simulink model "lin_hover_sim"  (R2025b)
settings: Solver=VariableStepAuto  StartTime=0.0  StopTime=t_sim  RelTol=1e-6  AbsTol=1e-6
values from neighbouring files (symbols this model uses):
  A = zeros(12,12)    [lin_hover.m]
  A_kfd = sys_kf_d.A    [lin_hover.m]
  Aomega = 1.00*Aref    (= 0.486439179934)    [lin_hover.m]    (also in non_lin_sim.m)
  Ax = 0.50*Aref    (= 0.243219589967)    [lin_hover.m]    (also in non_lin_sim.m)
  Ay = 0.50*Aref    (= 0.243219589967)    [lin_hover.m]    (also in non_lin_sim.m)
  Az = 0.35*Aref    (= 0.170253712977)    [lin_hover.m]    (also in non_lin_sim.m)
  B = zeros(12,4)    [lin_hover.m]
  B_kfd = sys_kf_d.B    [lin_hover.m]
  C11 = 4.58e-4    (= 0.000458)    [lin_hover.m]    (also in non_lin_sim.m)
  C21 = -.562    (= -0.562)    [lin_hover.m]    (also in non_lin_sim.m)
  CDw = 1.0    (= 1)    [lin_hover.m]    (also in non_lin_sim.m)
  CDx = 1.0    (= 1)    [lin_hover.m]    (also in non_lin_sim.m)
  CDy = 1.0    (= 1)    [lin_hover.m]    (also in non_lin_sim.m)
  CDz = 1.0    (= 1)    [lin_hover.m]    (also in non_lin_sim.m)
  g = 9.81    [lin_hover.m]    (also in non_lin_sim.m)
  Ix = I(1,1)    [lin_hover.m]    (also in non_lin_sim.m)
  Iy = I(2,2)    [lin_hover.m]    (also in non_lin_sim.m)
  Iz = I(3,3)    [lin_hover.m]    (also in non_lin_sim.m)
  k_tau = 0.00    (= 0)    [lin_hover.m]    (also in non_lin_sim.m)
  m = 0.110    (= 0.11)    [lin_hover.m]    (also in non_lin_sim.m)
  max_pot = 1950    [lin_hover.m]
  noise_true = 1    [lin_hover.m]
  pitch_D = 0    [lin_hover.m]
  pitch_I = 0.005*Iy/Ix    [lin_hover.m]
  pitch_P = 0.022*Iy/Ix    [lin_hover.m]
  rho = 1.225    [lin_hover.m]    (also in non_lin_sim.m)
  roll_D = 0    [lin_hover.m]
  roll_I = 0.005    [lin_hover.m]
  roll_P = 0.022    [lin_hover.m]
  S = 0.11    [lin_hover.m]    (also in non_lin_sim.m)
  seed = 23341    [lin_hover.m]
  sim_fidelity = 'high'    [lin_hover.m]
  strength = 50    [lin_hover.m]
  tau_wing = 0.1/2.2    (= 0.0454545454545)    [lin_hover.m]
  Ts = 1/fs    (= 0.00025)    [lin_hover.m]
  u0 = (m*g/4 - C21)/C11    (= 1816.10262009)    [lin_hover.m]
  X0 = zeros([12,1])    [lin_hover.m]
  Xref = zeros([12,1])    [lin_hover.m]
  Xu = rho*CDx*Ax*v_ref    (= 0.148971998855)    [lin_hover.m]    (also in non_lin_sim.m)
  yaw_D = 0    [lin_hover.m]
  yaw_I = 0.001    [lin_hover.m]
  yaw_P = 0.001    [lin_hover.m]
  Yv = rho*CDy*Ay*v_ref    (= 0.148971998855)    [lin_hover.m]    (also in non_lin_sim.m)
  Zw = rho*CDz*Az*w_ref    (= 0.104280399198)    [lin_hover.m]    (also in non_lin_sim.m)
undefined symbols (not defined in the file or in its folder): accel, C_kf, D_kf, DiscIntNeverNeededParam, Discrete, dspblkCoreblockFVToolHelper, gcbh, gyro, mahoney, R_kf, Time, x_kf0
libraries: slpidlib x5, simulink_extras x5, simulink x3, ctrlSharedLib x1
settings Model: Creator=bmatt  LastModifiedBy=bmatt
settings DebuggingCC: SignalInfNanChecking=error  SignalRangeChecking=error

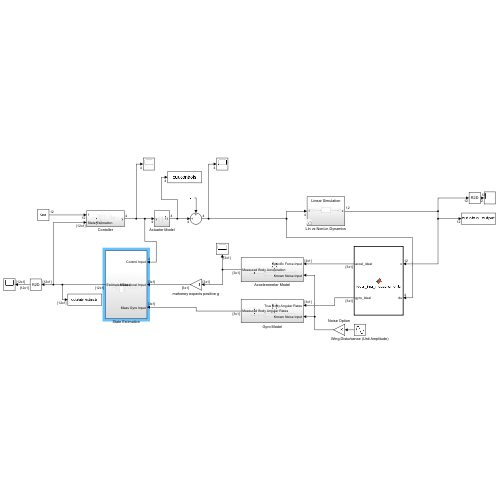
[thumbnail: Simulink's stored preview of the top-level diagram]
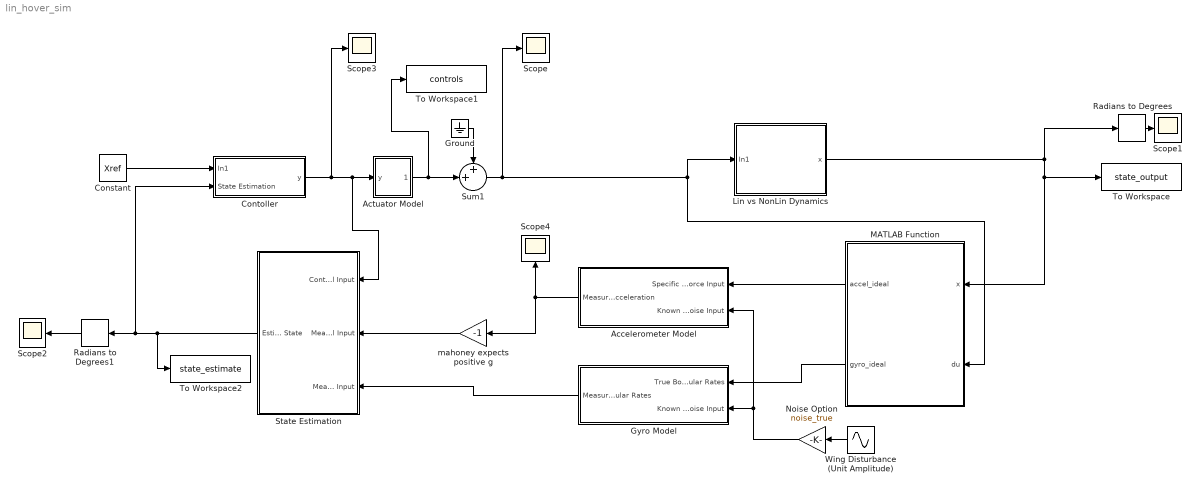
== system lin_hover_sim ==
  Accelerometer Model : Subsystem
  Actuator Model : Subsystem
  Constant : Constant  Value=Xref  SampleTime=-1
  Contoller : Subsystem
  Ground : Ground
  Gyro Model : Subsystem
  Lin vs NonLin Dynamics : Subsystem  Variant=on
  MATLAB Function : MATLAB Function  TreatAsAtomicUnit=on
  Noise Option : Gain  Gain=noise_true
  Radians to Degrees : simulink_extras/Transformations/Radians to Degrees
  Radians to Degrees1 : simulink_extras/Transformations/Radians to Degrees
  Scope{,1..4} (5 alike) : Scope
      Scope settings: ActiveDisplayYMinimum=-18.295353079019556  ActiveDisplayYMaximum=14.608808990960183
      Scope1 settings: ActiveDisplayYMinimum=-57.493316939596269  ActiveDisplayYMaximum=14.428367766901045
      Scope2 settings: ActiveDisplayYMinimum=-37.103950229220729  ActiveDisplayYMaximum=16.0841911942195  DataLoggingVariableName=ScopeData2
      Scope3 settings: ActiveDisplayYMinimum=-1  ActiveDisplayYMaximum=1  DataLoggingVariableName=ScopeData9
      Scope4 settings: ActiveDisplayYMinimum=-26.796825567144111  ActiveDisplayYMaximum=14.82950437821362  DataLoggingVariableName=ScopeData10
  State Estimation : Subsystem
  Sum1 : Sum  Inputs=++|
  To Workspace : ToWorkspace  VariableName=state_output  SaveFormat=Structure With Time  SampleTime=-1
  To Workspace1 : ToWorkspace  VariableName=controls  SaveFormat=Structure With Time  SampleTime=-1
  To Workspace2 : ToWorkspace  VariableName=state_estimate  SaveFormat=Structure With Time  SampleTime=-1
  Wing Disturbance (Unit Amplitude) : Sin  Frequency=2*pi*24  SampleTime=0
  mahoney expects positive g : Gain  Gain=-1
  wires:
  Sum1/1 -> Scope/1, Lin vs NonLin Dynamics/1(In1), MATLAB Function/2(du)
  Constant/1 -> Contoller/1(In1)
  Contoller/1(y) -> Actuator Model/1(y), State Estimation/1(Control Input), Scope3/1
  Actuator Model/1(Out1) -> Sum1/2, To Workspace1/1
  State Estimation/1(Estimated State) -> To Workspace2/1, Contoller/2(State Estimation), Radians to Degrees1/1
  Ground/1 -> Sum1/1
  Radians to Degrees/1 -> Scope1/1
  Radians to Degrees1/1 -> Scope2/1
  Accelerometer Model/1(Measured Body Acceleration) -> mahoney expects positive g/1, Scope4/1
  Gyro Model/1(Measured Body Angular Rates) -> State Estimation/3(Meas Gyro Input)
  MATLAB Function/1(accel_ideal) -> Accelerometer Model/1(Specific Force Input)
  MATLAB Function/2(gyro_ideal) -> Gyro Model/1(True Body Angular Rates)
  mahoney expects positive g/1 -> State Estimation/2(Meas Accel Input)
  Wing Disturbance (Unit Amplitude)/1 -> Noise Option/1
  Noise Option/1 -> Accelerometer Model/2(Known Noise Input), Gyro Model/2(Known Noise Input)
  Lin vs NonLin Dynamics/1(x) -> To Workspace/1, MATLAB Function/1(x), Radians to Degrees/1

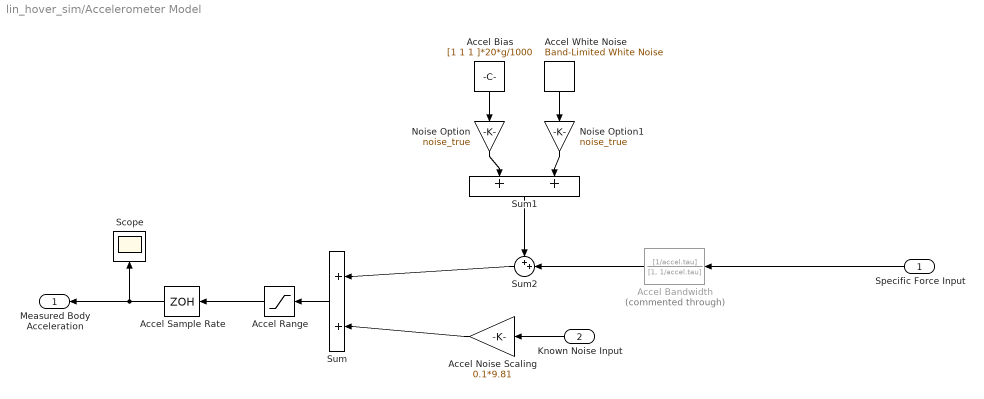
== system lin_hover_sim/Accelerometer Model ==
  Specific Force Input : Inport
  Known Noise Input : Inport  Port=2
  Accel White Noise : simulink/Sources/Band-Limited White Noise  Cov=[1 1 1]*((0.16*9.81/1000)*sqrt(740))^2  Ts=1/1600  seed=[seed]
  Accel Bandwidth : DiscreteTransferFcn  Commented=through  LoadFcn=dspblkCoreblockFVToolHelper(gcbh,'load');  Numerator=[1/accel.tau]  Denominator=[1, 1/accel.tau]
      settings: CopyFcn=dspblkCoreblockFVToolHelper(gcbh,'copy');  DeleteFcn=dspblkCoreblockFVToolHelper(gcbh,'close');  ModelCloseFcn=dspblkCoreblockFVToolHelper(gcbh,'close');  PreSaveFcn=dspblkCoreblockFVToolHelper(gcbh,'presave');  PostSaveFcn=dspblkCoreblockFVToolHelper(gcbh,'postsave');  CloseFcn=dspblkCoreblockFVToolHelper(gcbh,'close');
  Accel Bias : Constant  Value=[1 1 1 ]*20*g/1000  SampleTime=1/1600
  Accel Noise Scaling : Gain  Gain=0.1*9.81
  Accel Range : Saturate  UpperLimit=4*9.81  LowerLimit=-4*9.81
  Accel Sample Rate : ZeroOrderHold  SampleTime=1/1600
  Noise Option : Gain  Gain=noise_true
  Noise Option1 : Gain  Gain=noise_true
  Scope : Scope
      settings: ActiveDisplayYMinimum=-33.285329290238963  ActiveDisplayYMaximum=9.7506326968606309  DataLoggingVariableName=ScopeData13
  Sum : Sum  Inputs=+|+
  Sum1 : Sum  Inputs=+|+
  Sum2 : Sum  Inputs=++|
  Measured Body Acceleration : Outport
  wires:
  Sum/1 -> Accel Range/1
  Sum2/1 -> Sum/1
  Accel Sample Rate/1 -> Scope/1, Measured Body Acceleration/1
  Known Noise Input/1 -> Accel Noise Scaling/1
  Accel Bandwidth/1 -> Sum2/2
  Specific Force Input/1 -> Accel Bandwidth/1
  Sum1/1 -> Sum2/1
  Accel Noise Scaling/1 -> Sum/2
  Accel Range/1 -> Accel Sample Rate/1
  Noise Option/1 -> Sum1/1
  Accel Bias/1 -> Noise Option/1
  Noise Option1/1 -> Sum1/2
  Accel White Noise/1 -> Noise Option1/1

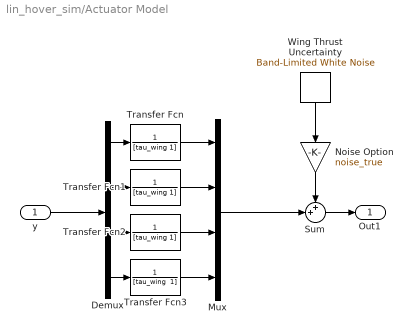
== system lin_hover_sim/Actuator Model ==
  y : Inport
  Demux : Demux
  Mux : Mux
  Noise Option : Gain  Gain=noise_true
  Sum : Sum  Inputs=++|
  Transfer Fcn : TransferFcn  Denominator=[tau_wing 1]
  Transfer Fcn1 : TransferFcn  Denominator=[tau_wing 1]
  Transfer Fcn2 : TransferFcn  Denominator=[tau_wing 1]
  Transfer Fcn3 : TransferFcn  Denominator="[tau_wing  1]"
  Wing Thrust Uncertainty : simulink/Sources/Band-Limited White Noise  Cov=1*[0.000001566122567;0.000001566122567;0.000001566122567;0.000001566122567]  Ts=Ts  seed=[seed]
  Out1 : Outport
  wires:
  Demux/4 -> Transfer Fcn3/1
  Demux/1 -> Transfer Fcn/1
  Demux/2 -> Transfer Fcn1/1
  Demux/3 -> Transfer Fcn2/1
  Transfer Fcn/1 -> Mux/1
  Transfer Fcn1/1 -> Mux/2
  Transfer Fcn2/1 -> Mux/3
  Transfer Fcn3/1 -> Mux/4
  y/1 -> Demux/1
  Sum/1 -> Out1/1
  Mux/1 -> Sum/2
  Wing Thrust Uncertainty/1 -> Noise Option/1
  Noise Option/1 -> Sum/1

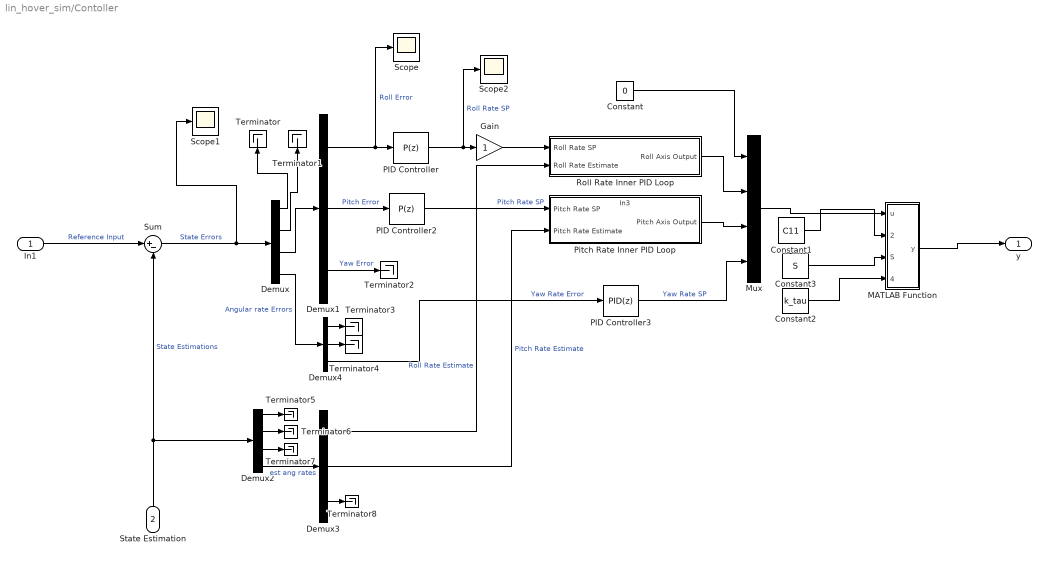
== system lin_hover_sim/Contoller ==
  In1 : Inport
  State Estimation : Inport  Port=2
  Constant : Constant  Value=0
  Constant1 : Constant  Value=C11
  Constant2 : Constant  Value=k_tau
  Constant3 : Constant  Value=S
  Demux : Demux  Outputs=[3 3 3 3]
  Demux1 : Demux  Outputs=[1 1 1]
  Demux2 : Demux  Outputs=[3 3 3 3]
  Demux3 : Demux  Outputs=[1 1 1]
  Demux4 : Demux  Outputs=[1 1 1]
  Gain : Gain
  MATLAB Function : MATLAB Function  TreatAsAtomicUnit=on
  Mux : Mux
  PID Controller : slpidlib/PID Controller  Controller=P  Form=Parallel  TimeDomain=Discrete-time  UseExternalTs=off  SampleTime=Ts  IntegratorMethod=Forward Euler  FilterMethod=Forward Euler  ControllerParametersSource=internal  P=strength/10  I=194.232873086371  UseKiTs=off  D=-0.0894221705749344  UseExternalDerivativeSource=off  N=55.5911819026225  UseFilter=on  TunerSelectOption=Frequency Response Based  InitialConditionSource=internal  InitialConditionForIntegrator=Xref(7) - X0(7)  InitialConditionForFilter=0  DifferentiatorICPrevScaledInput=0  ExternalReset=none  TrackingMode=off  Kt=1  LimitOutput=on  SatLimitsSource=internal  UpperSaturationLimit=3.5  LowerSaturationLimit=-3.5  LinearizeAsGain=on  AntiWindupMode=external  Kb=1  LimitIntegrator=off  UpperIntegratorSaturationLimit=inf  LowerIntegratorSaturationLimit=-inf  POutMin=[]  POutMax=[]  IOutMin=[]  IOutMax=[]  DOutMin=[]  DOutMax=[]  NOutMin=[]  NOutMax=[]  SumOutMin=[]  SumOutMax=[]  SaturationOutMin=[]  SaturationOutMax=[]  PParamMin=[]  PParamMax=[]  IParamMin=[]  IParamMax=[]  DParamMin=[]  DParamMax=[]  NParamMin=[]  NParamMax=[]  KbParamMin=[]  KbParamMax=[]  KtParamMin=[]  KtParamMax=[]  KbOutMin=[]  KbOutMax=[]  KtOutMin=[]  KtOutMax=[]  IntegratorOutMin=[]  IntegratorOutMax=[]  FilterOutMin=[]  FilterOutMax=[]  SumI1OutMin=[]  SumI1OutMax=[]  SumI2OutMin=[]  SumI2OutMax=[]  SumI3OutMin=[]  SumI3OutMax=[]  SumI4OutMin=[]  SumI4OutMax=[]  SumDOutMin=[]  SumDOutMax=[]  DifferentiatorOutMin=[]  DifferentiatorOutMax=[]  FilterDiffOutCoefMin=[]  FilterDiffOutCoefMax=[]  ReciprocalOutMin=[]  ReciprocalOutMax=[]  SumDenOutMin=[]  SumDenOutMax=[]  SumNumOutMin=[]  SumNumOutMax=[]  DivideOutMin=[]  DivideOutMax=[]  UdiffTsProdOutMin=[]  UdiffTsProdOutMax=[]  NTsProdOutMin=[]  NTsProdOutMax=[]  UintegralTsProdOutMin=[]  UintegralTsProdOutMax=[]  UngainTsProdOutMin=[]  UngainTsProdOutMax=[]  ClampingZeroOutDataTypeStr=Inherit: Inherit via back propagation  ClampingZeroOutMin=[]  ClampingZeroOutMax=[]  FilterDenConstantOutDataTypeStr=Inherit: Inherit via back propagation  FilterDenConstantOutMin=[]  FilterDenConstantOutMax=[]  PCopyOutDataTypeStr=Inherit: Inherit via back propagation  PCopyOutMin=[]  PCopyOutMax=[]  NCopyOutDataTypeStr=Inherit: Inherit via back propagation  NCopyOutMin=[]  NCopyOutMax=[]  IntegratorContinuousStateAttributes=''  IntegratorStateMustResolveToSignalObject=off  IntegratorRTWStateStorageClass=Auto  FilterContinuousStateAttributes=''  FilterStateMustResolveToSignalObject=off  FilterRTWStateStorageClass=Auto  ParallelPVariant=InternalParameters  IdealPVariant=Disabled  IVariant=Disabled  DVariant=Disabled  IntegratorVariant=Disabled  SatVariant=Enabled  AWVariant=Disabled  PCopyVariant=Disabled  TRVariant=Disabled  FdbkBlocksVariant=Forward  IdealPFdbkVariant=Disabled  SatFdbkVariant=Disabled  DerivativeFilterVariant=Disabled  NVariant=Disabled  NCopyVariant=Disabled_SignalSpec  FilterICVariant=Disabled  IntegratorICVariant=Disabled  ExternalResetVariant=Disabled  TRSumVariant=Passthrough  SumFdbkVariant=Disabled  SumVariant=Passthrough_P  TsampFilterVariant=InternalTs  TsampNgainVariant=Passthrough  TsampIntegralVariant=Disabled_SignalSpec  ExternalSaturationOutDataTypeStr=Inherit: Same as second input  DerivativeSourceVariant=Disabled  PreIntVariant=InternalPreInt
  PID Controller2 : slpidlib/PID Controller  Controller=P  Form=Parallel  TimeDomain=Discrete-time  UseExternalTs=off  SampleTime=Ts  IntegratorMethod=Forward Euler  FilterMethod=Forward Euler  ControllerParametersSource=internal  P=strength/10  I=0.287608182877056  UseKiTs=off  D=0  UseExternalDerivativeSource=off  N=100  UseFilter=on  TunerSelectOption=Transfer Function Based (PID Tuner App)  InitialConditionSource=internal  InitialConditionForIntegrator=Xref(8) - X0(8)  InitialConditionForFilter=0  DifferentiatorICPrevScaledInput=0  ExternalReset=none  TrackingMode=off  Kt=1  LimitOutput=on  SatLimitsSource=internal  UpperSaturationLimit=3.5  LowerSaturationLimit=-3.5  LinearizeAsGain=off  AntiWindupMode=none  Kb=1  LimitIntegrator=off  UpperIntegratorSaturationLimit=inf  LowerIntegratorSaturationLimit=-inf  POutMin=[]  POutMax=[]  IOutMin=[]  IOutMax=[]  DOutMin=[]  DOutMax=[]  NOutMin=[]  NOutMax=[]  SumOutMin=[]  SumOutMax=[]  SaturationOutMin=[]  SaturationOutMax=[]  PParamMin=[]  PParamMax=[]  IParamMin=[]  IParamMax=[]  DParamMin=[]  DParamMax=[]  NParamMin=[]  NParamMax=[]  KbParamMin=[]  KbParamMax=[]  KtParamMin=[]  KtParamMax=[]  KbOutMin=[]  KbOutMax=[]  KtOutMin=[]  KtOutMax=[]  IntegratorOutMin=[]  IntegratorOutMax=[]  FilterOutMin=[]  FilterOutMax=[]  SumI1OutMin=[]  SumI1OutMax=[]  SumI2OutMin=[]  SumI2OutMax=[]  SumI3OutMin=[]  SumI3OutMax=[]  SumI4OutMin=[]  SumI4OutMax=[]  SumDOutMin=[]  SumDOutMax=[]  DifferentiatorOutMin=[]  DifferentiatorOutMax=[]  FilterDiffOutCoefMin=[]  FilterDiffOutCoefMax=[]  ReciprocalOutMin=[]  ReciprocalOutMax=[]  SumDenOutMin=[]  SumDenOutMax=[]  SumNumOutMin=[]  SumNumOutMax=[]  DivideOutMin=[]  DivideOutMax=[]  UdiffTsProdOutMin=[]  UdiffTsProdOutMax=[]  NTsProdOutMin=[]  NTsProdOutMax=[]  UintegralTsProdOutMin=[]  UintegralTsProdOutMax=[]  UngainTsProdOutMin=[]  UngainTsProdOutMax=[]  ClampingZeroOutDataTypeStr=Inherit: Inherit via back propagation  ClampingZeroOutMin=[]  ClampingZeroOutMax=[]  FilterDenConstantOutDataTypeStr=Inherit: Inherit via back propagation  FilterDenConstantOutMin=[]  FilterDenConstantOutMax=[]  PCopyOutDataTypeStr=Inherit: Inherit via back propagation  PCopyOutMin=[]  PCopyOutMax=[]  NCopyOutDataTypeStr=Inherit: Inherit via back propagation  NCopyOutMin=[]  NCopyOutMax=[]  IntegratorContinuousStateAttributes=''  IntegratorStateMustResolveToSignalObject=off  IntegratorRTWStateStorageClass=Auto  FilterContinuousStateAttributes=''  FilterStateMustResolveToSignalObject=off  FilterRTWStateStorageClass=Auto  ParallelPVariant=InternalParameters  IdealPVariant=Disabled  IVariant=Disabled  DVariant=Disabled  IntegratorVariant=Disabled  SatVariant=Enabled  AWVariant=Disabled  PCopyVariant=Disabled  TRVariant=Disabled  FdbkBlocksVariant=Forward  IdealPFdbkVariant=Disabled  SatFdbkVariant=Disabled  DerivativeFilterVariant=Disabled  NVariant=Disabled  NCopyVariant=Disabled_SignalSpec  FilterICVariant=Disabled  IntegratorICVariant=Disabled  ExternalResetVariant=Disabled  TRSumVariant=Passthrough  SumFdbkVariant=Disabled  SumVariant=Passthrough_P  TsampFilterVariant=InternalTs  TsampNgainVariant=Passthrough  TsampIntegralVariant=Disabled_SignalSpec  ExternalSaturationOutDataTypeStr=Inherit: Same as second input  DerivativeSourceVariant=Disabled  PreIntVariant=InternalPreInt
  PID Controller3 : slpidlib/PID Controller  Controller=PID  Form=Parallel  TimeDomain=Discrete-time  UseExternalTs=off  SampleTime=Ts  IntegratorMethod=Forward Euler  FilterMethod=Forward Euler  ControllerParametersSource=internal  P=yaw_P  I=yaw_I  UseKiTs=off  D=yaw_D  UseExternalDerivativeSource=off  N=44.2614212635521  UseFilter=on  TunerSelectOption=Transfer Function Based (PID Tuner App)  InitialConditionSource=internal  InitialConditionForIntegrator=Xref(12) - X0(12)  InitialConditionForFilter=0  DifferentiatorICPrevScaledInput=0  ExternalReset=none  TrackingMode=off  Kt=1  LimitOutput=on  SatLimitsSource=internal  UpperSaturationLimit=50  LowerSaturationLimit=-50  LinearizeAsGain=on  AntiWindupMode=clamping  Kb=1  LimitIntegrator=off  UpperIntegratorSaturationLimit=inf  LowerIntegratorSaturationLimit=-inf  POutMin=[]  POutMax=[]  IOutMin=[]  IOutMax=[]  DOutMin=[]  DOutMax=[]  NOutMin=[]  NOutMax=[]  SumOutMin=[]  SumOutMax=[]  SaturationOutMin=[]  SaturationOutMax=[]  PParamMin=[]  PParamMax=[]  IParamMin=[]  IParamMax=[]  DParamMin=[]  DParamMax=[]  NParamMin=[]  NParamMax=[]  KbParamMin=[]  KbParamMax=[]  KtParamMin=[]  KtParamMax=[]  KbOutMin=[]  KbOutMax=[]  KtOutMin=[]  KtOutMax=[]  IntegratorOutMin=[]  IntegratorOutMax=[]  FilterOutMin=[]  FilterOutMax=[]  SumI1OutMin=[]  SumI1OutMax=[]  SumI2OutMin=[]  SumI2OutMax=[]  SumI3OutMin=[]  SumI3OutMax=[]  SumI4OutMin=[]  SumI4OutMax=[]  SumDOutMin=[]  SumDOutMax=[]  DifferentiatorOutMin=[]  DifferentiatorOutMax=[]  FilterDiffOutCoefMin=[]  FilterDiffOutCoefMax=[]  ReciprocalOutMin=[]  ReciprocalOutMax=[]  SumDenOutMin=[]  SumDenOutMax=[]  SumNumOutMin=[]  SumNumOutMax=[]  DivideOutMin=[]  DivideOutMax=[]  UdiffTsProdOutMin=[]  UdiffTsProdOutMax=[]  NTsProdOutMin=[]  NTsProdOutMax=[]  UintegralTsProdOutMin=[]  UintegralTsProdOutMax=[]  UngainTsProdOutMin=[]  UngainTsProdOutMax=[]  ClampingZeroOutDataTypeStr=Inherit: Inherit via back propagation  ClampingZeroOutMin=[]  ClampingZeroOutMax=[]  FilterDenConstantOutDataTypeStr=Inherit: Inherit via back propagation  FilterDenConstantOutMin=[]  FilterDenConstantOutMax=[]  PCopyOutDataTypeStr=Inherit: Inherit via back propagation  PCopyOutMin=[]  PCopyOutMax=[]  NCopyOutDataTypeStr=Inherit: Inherit via back propagation  NCopyOutMin=[]  NCopyOutMax=[]  IntegratorContinuousStateAttributes=''  IntegratorStateMustResolveToSignalObject=off  IntegratorRTWStateStorageClass=Auto  FilterContinuousStateAttributes=''  FilterStateMustResolveToSignalObject=off  FilterRTWStateStorageClass=Auto  ParallelPVariant=InternalParameters  IdealPVariant=Disabled  IVariant=InternalParameters  DVariant=InternalParameters  IntegratorVariant=Discrete  SatVariant=Enabled  AWVariant=DiscClampingParallel  PCopyVariant=Disabled  TRVariant=Disabled  FdbkBlocksVariant=Forward  IdealPFdbkVariant=Disabled  SatFdbkVariant=Disabled  DerivativeFilterVariant=ForwardEulerFilter  NVariant=InternalParameters  NCopyVariant=Disabled  FilterICVariant=InternalICsFilter  IntegratorICVariant=InternalICs  ExternalResetVariant=Disabled  TRSumVariant=Passthrough  SumFdbkVariant=Disabled  SumVariant=Sum_PID  TsampFilterVariant=InternalTs  TsampNgainVariant=Passthrough  TsampIntegralVariant=Disabled_SignalSpec  ExternalSaturationOutDataTypeStr=Inherit: Same as second input  DerivativeSourceVariant=ErrorSignal  PreIntVariant=InternalPreInt
  Pitch Rate Inner PID Loop : Subsystem
      settings: PortSchema="{\"entries\":[{\"content\":{\"sides\":[{\"content\":{\"connectorIds\":[\"In1\",\"In2\"]},\"type\":\"ConnectorPlacement.EquallySpacedRectSide\",\"uuid\":\"55092445-7ee8-4ffe-8f8b-ed2279b4bdff\"},{\"content\":{\"connectorIds\":[\"Out1\"],\"side\":\"RIGHT\"},\"type\":\"ConnectorPlacement.EquallySpacedRectSide\",\"uuid\":\"8c2bc3dc-27c0-44be-8f47-54c9e25a8d58\"},{\"content\":{\"connectorIds\":[\"In3\"],\"side\":\"TOP\"},\"type\":\"ConnectorPlacement.EquallySpacedRectSide\",\"uuid\":\"397705a7-8291-491e-a33c-c005fef1c916\"}]},\"type\":\"ConnectorPlacement.EquallySpacedConnector\",\"uuid\":\"53948e4d-9aad-44a3-9c6c-86850b479a5f\"}],\"packageUris\":[\"http://schema.mathworks.com/mf0/Connector/R2020b\"],\"version\":\"1.0\"}"
  Roll Rate Inner PID Loop : Subsystem
  Scope : Scope
      settings: ActiveDisplayYMinimum=-1  ActiveDisplayYMaximum=1  DataLoggingVariableName=ScopeData3
  Scope1 : Scope
      settings: ActiveDisplayYMinimum=-19.957380874165978  ActiveDisplayYMaximum=76.260116876327913  DataLoggingVariableName=ScopeData4
  Scope2 : Scope
      settings: ActiveDisplayYMinimum=-1.9310995592786648  ActiveDisplayYMaximum=0.59639946586768922  DataLoggingVariableName=ScopeData6
  Sum : Sum  Inputs=|+-
  Terminator{,1..8} (9 alike) : Terminator
  y : Outport
  wires:
  In1/1 -> Sum/1  "Reference Input"
  State Estimation/1 -> Demux2/1, Sum/2  "State Estimations"
  Sum/1 -> Scope1/1, Demux/1  "State Errors"
  Demux/3 -> Demux1/1
  Demux2/4 -> Demux3/1  "est ang rates"
  Demux1/2 -> PID Controller2/1  "Pitch Error"
  Demux3/1 -> Roll Rate Inner PID Loop/2(Roll Rate Estimate)  "Roll Rate Estimate"
  PID Controller2/1 -> Pitch Rate Inner PID Loop/1(Pitch Rate SP)  "Pitch Rate SP"
  Demux3/2 -> Pitch Rate Inner PID Loop/2(Pitch Rate Estimate)  "Pitch Rate Estimate"
  Demux/4 -> Demux4/1  "Angular rate Errors"
  Demux4/3 -> PID Controller3/1  "Yaw Rate Error"
  Roll Rate Inner PID Loop/1(Roll Axis Output) -> Mux/2
  Pitch Rate Inner PID Loop/1(Pitch Axis Output) -> Mux/3
  PID Controller3/1 -> Mux/4  "Yaw Rate SP"
  Demux/1 -> Terminator/1
  Demux/2 -> Terminator1/1
  Demux1/3 -> Terminator2/1  "Yaw Error"
  Demux4/1 -> Terminator3/1
  Demux4/2 -> Terminator4/1
  Demux2/1 -> Terminator5/1
  Demux2/2 -> Terminator6/1
  Demux2/3 -> Terminator7/1
  Demux3/3 -> Terminator8/1
  Demux1/1 -> Scope/1, PID Controller/1  "Roll Error"
  Constant/1 -> Mux/1
  Mux/1 -> MATLAB Function/1(u)
  Constant1/1 -> MATLAB Function/2(C11)
  Constant2/1 -> MATLAB Function/4(k_tau)
  Constant3/1 -> MATLAB Function/3(S)
  PID Controller/1 -> Scope2/1, Gain/1  "Roll Rate SP"
  Gain/1 -> Roll Rate Inner PID Loop/1(Roll Rate SP)
  MATLAB Function/1(y) -> y/1

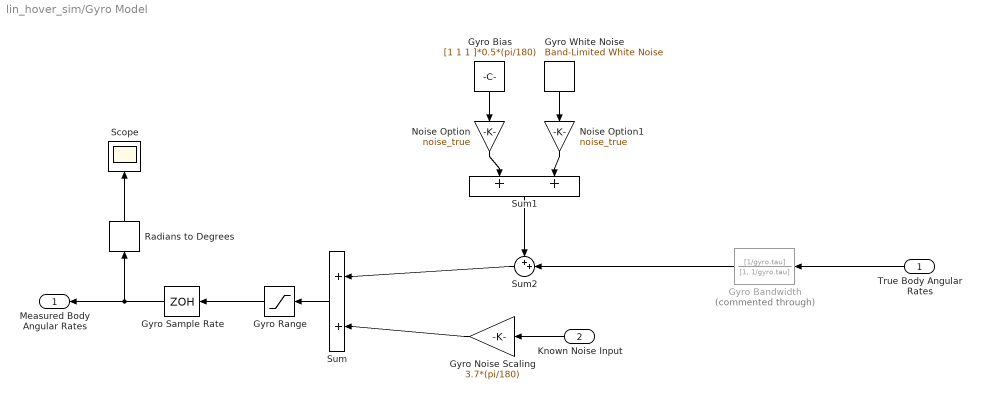
== system lin_hover_sim/Gyro Model ==
  True Body Angular Rates : Inport
  Known Noise Input : Inport  Port=2
  Gyro White Noise : simulink/Sources/Band-Limited White Noise  Cov=[1 1 1]*(0.007*(pi/180)*sqrt(751))^2  Ts=1/3200  seed=[seed]
  Gyro Bandwidth : DiscreteTransferFcn  Commented=through  LoadFcn=dspblkCoreblockFVToolHelper(gcbh,'load');  Numerator=[1/gyro.tau]  Denominator=[1, 1/gyro.tau]
      settings: CopyFcn=dspblkCoreblockFVToolHelper(gcbh,'copy');  DeleteFcn=dspblkCoreblockFVToolHelper(gcbh,'close');  ModelCloseFcn=dspblkCoreblockFVToolHelper(gcbh,'close');  PreSaveFcn=dspblkCoreblockFVToolHelper(gcbh,'presave');  PostSaveFcn=dspblkCoreblockFVToolHelper(gcbh,'postsave');  CloseFcn=dspblkCoreblockFVToolHelper(gcbh,'close');
  Gyro Bias : Constant  Value=[1 1 1 ]*0.5*(pi/180)  SampleTime=1/3200
  Gyro Noise Scaling : Gain  Gain=3.7*(pi/180)
  Gyro Range : Saturate  UpperLimit=1000*(pi/180)  LowerLimit=-1000*(pi/180)
  Gyro Sample Rate : ZeroOrderHold  SampleTime=1/3200
  Noise Option : Gain  Gain=noise_true
  Noise Option1 : Gain  Gain=noise_true
  Radians to Degrees : simulink_extras/Transformations/Radians to Degrees
  Scope : Scope
      settings: ActiveDisplayYMinimum=-95.458388464877785  ActiveDisplayYMaximum=62.296372418802648  DataLoggingVariableName=ScopeData14
  Sum : Sum  Inputs=+|+
  Sum1 : Sum  Inputs=+|+
  Sum2 : Sum  Inputs=++|
  Measured Body Angular Rates : Outport
  wires:
  True Body Angular Rates/1 -> Gyro Bandwidth/1
  Sum/1 -> Gyro Range/1
  Known Noise Input/1 -> Gyro Noise Scaling/1
  Sum1/1 -> Sum2/1
  Gyro Bandwidth/1 -> Sum2/2
  Gyro Sample Rate/1 -> Radians to Degrees/1, Measured Body Angular Rates/1
  Gyro Range/1 -> Gyro Sample Rate/1
  Sum2/1 -> Sum/1
  Gyro Noise Scaling/1 -> Sum/2
  Noise Option/1 -> Sum1/1
  Gyro Bias/1 -> Noise Option/1
  Gyro White Noise/1 -> Noise Option1/1
  Noise Option1/1 -> Sum1/2
  Radians to Degrees/1 -> Scope/1

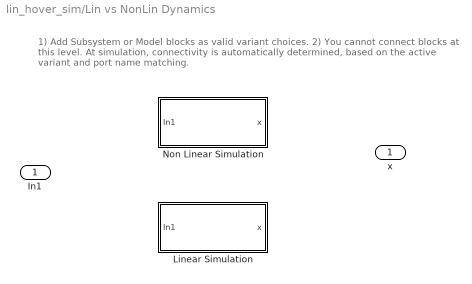
== system lin_hover_sim/Lin vs NonLin Dynamics ==
  note: 1) Add Subsystem or Model blocks as valid variant choices.
      | 2) You cannot connect blocks at this level. At simulation, connectivity is automatically
      | determined, based on the active variant and port name matching.
  In1 : Inport
  Linear Simulation : Subsystem  VariantControl=strcmp(sim_fidelity,'low')
  Non Linear Simulation : Subsystem  VariantControl=strcmp(sim_fidelity,'high')
  x : Outport

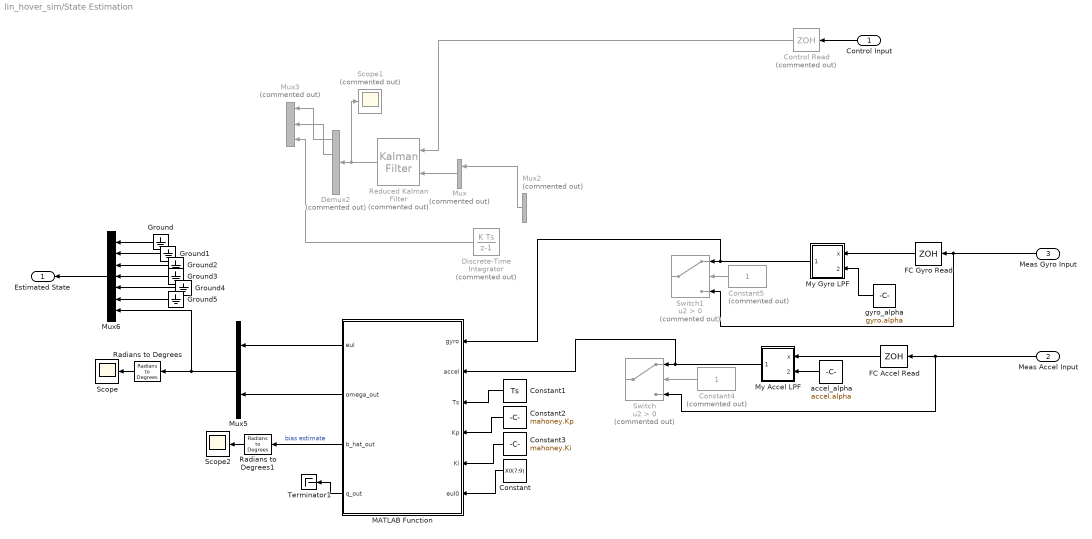
== system lin_hover_sim/State Estimation ==
  Control Input : Inport
  Meas Accel Input : Inport  Port=2
  Meas Gyro Input : Inport  Port=3
  Constant : Constant  Value=X0(7:9)
  Constant1 : Constant  Value=Ts
  Constant2 : Constant  Value=mahoney.Kp
  Constant3 : Constant  Value=mahoney.Ki
  Constant4 : Constant  Commented=on
  Constant5 : Constant  Commented=on
  Control Read : ZeroOrderHold  Commented=on  SampleTime=Ts
  Demux2 : Demux  Commented=on  Outputs=[1 1 1 1]
  Discrete-Time Integrator : DiscreteIntegrator  Commented=on  InitialCondition=X0(9)  SampleTime=-1  ICPrevOutput=DiscIntNeverNeededParam  ICPrevScaledInput=DiscIntNeverNeededParam
  FC Accel Read : ZeroOrderHold  SampleTime=Ts
  FC Gyro Read : ZeroOrderHold  SampleTime=Ts
  Ground{,1..5} (6 alike) : Ground
  MATLAB Function : MATLAB Function  TreatAsAtomicUnit=on
  Mux : Mux  Commented=on  Inputs=2
  Mux2 : Mux  Commented=on  Inputs=2
  Mux3 : Mux  Commented=on  Inputs=3
  Mux5 : Mux  Inputs=2
  Mux6 : Mux  Inputs=7
  My Accel LPF : MATLAB Function  TreatAsAtomicUnit=on
  My Gyro LPF : MATLAB Function  TreatAsAtomicUnit=on
  Radians to Degrees : simulink_extras/Transformations/Radians to Degrees
  Radians to Degrees1 : simulink_extras/Transformations/Radians to Degrees
  Reduced Kalman Filter : ctrlSharedLib/Kalman Filter  Commented=on  TimeDomain=Discrete-Time  UseCurrentEstimator=on  ModelSource=Individual A, B, C, D matrices  ModelSourceVariable=ss(0.95,1,1,0,1)  A=A_kfd  B=B_kfd  C=C_kf  D=D_kf  NumberOfStates=1  NumberOfInputs=1  NumberOfOutputs=1  InitialEstimateSource=Dialog  X0=x_kf0  P0=10  UseK=off  UseGH=off  NumberOfProcessNoiseInputs=1  G=1  TimeInvariantG=on  H=0  TimeInvariantH=on  Q=Q_kf  TimeInvariantQ=on  R=R_kf  TimeInvariantR=on  N=0  TimeInvariantN=on  AddInputPort=on  AddEnablePort=off  OutputEstimatedY=off  OutputP=off  Ts=Ts
  Scope : Scope
      settings: ActiveDisplayYMinimum=-26.089425701954106  ActiveDisplayYMaximum=28.420657491696105  DataLoggingVariableName=ScopeData11
  Scope1 : Scope  Commented=on
      settings: ActiveDisplayYMinimum=-1.3309196424589129  ActiveDisplayYMaximum=1.1359717359097128  DataLoggingVariableName=ScopeData12
  Scope2 : Scope
      settings: ActiveDisplayYMinimum=-22.985912454818191  ActiveDisplayYMaximum=12.151773195582674  DataLoggingVariableName=ScopeData15
  Switch : Switch  Commented=on  Criteria=u2 > Threshold  SaturateOnIntegerOverflow=off  InputSameDT=off
  Switch1 : Switch  Commented=on  Criteria=u2 > Threshold  SaturateOnIntegerOverflow=off  InputSameDT=off
  Terminator1 : Terminator
  accel_alpha : Constant  Value=accel.alpha
  gyro_alpha : Constant  Value=gyro.alpha
  Estimated State : Outport
  wires:
  Meas Gyro Input/1 -> Switch1/3, FC Gyro Read/1
  Meas Accel Input/1 -> FC Accel Read/1, Switch/3
  Mux/1 -> Reduced Kalman Filter/2
  Control Input/1 -> Control Read/1
  FC Gyro Read/1 -> My Gyro LPF/1(x)
  Reduced Kalman Filter/1 -> Scope1/1, Demux2/1
  Demux2/1 -> Mux3/1
  Demux2/2 -> Mux3/2
  Mux5/1 -> Mux6/7, Radians to Degrees/1
  Control Read/1 -> Reduced Kalman Filter/1
  Mux2/1 -> Mux/1
  Mux6/1 -> Estimated State/1
  Ground/1 -> Mux6/1
  Ground1/1 -> Mux6/2
  Ground2/1 -> Mux6/3
  Ground3/1 -> Mux6/4
  Ground4/1 -> Mux6/5
  Ground5/1 -> Mux6/6
  gyro_alpha/1 -> My Gyro LPF/2(gyro_alpha)
  FC Accel Read/1 -> My Accel LPF/1(x)
  My Accel LPF/1(xlpf) -> MATLAB Function/2(accel), Switch/1
  MATLAB Function/1(eul) -> Mux5/1
  Discrete-Time Integrator/1 -> Mux3/3
  Constant1/1 -> MATLAB Function/3(Ts)
  accel_alpha/1 -> My Accel LPF/2(accel_alpha)
  Constant/1 -> MATLAB Function/6(eul0)
  Constant2/1 -> MATLAB Function/4(Kp)
  Constant3/1 -> MATLAB Function/5(Ki)
  MATLAB Function/3(b_hat_out) -> Radians to Degrees1/1  "bias estimate"
  MATLAB Function/4(q_out) -> Terminator1/1
  MATLAB Function/2(omega_out) -> Mux5/2
  Radians to Degrees/1 -> Scope/1
  Radians to Degrees1/1 -> Scope2/1
  Constant4/1 -> Switch/2
  Constant5/1 -> Switch1/2
  My Gyro LPF/1(xlpf) -> MATLAB Function/1(gyro), Switch1/1

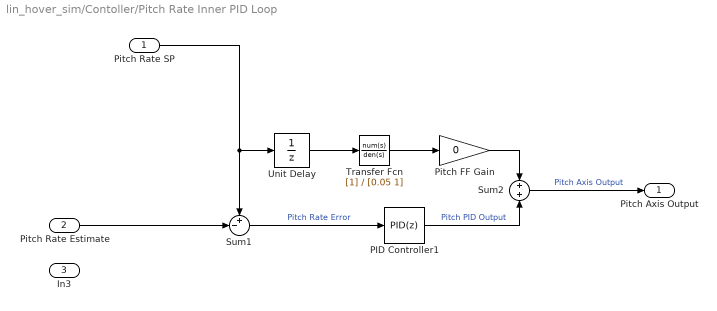
== system lin_hover_sim/Contoller/Pitch Rate Inner PID Loop ==
  Pitch Rate SP : Inport
  Pitch Rate Estimate : Inport  Port=2
  In3 : Inport  Port=3
  PID Controller1 : slpidlib/PID Controller  Controller=PID  Form=Parallel  TimeDomain=Discrete-time  UseExternalTs=off  SampleTime=Ts  IntegratorMethod=Forward Euler  FilterMethod=Forward Euler  ControllerParametersSource=internal  P=pitch_P  I=pitch_I  UseKiTs=off  D=pitch_D  UseExternalDerivativeSource=off  N=40  UseFilter=on  TunerSelectOption=Transfer Function Based (PID Tuner App)  InitialConditionSource=internal  InitialConditionForIntegrator=Xref(11) - X0(11)  InitialConditionForFilter=0  DifferentiatorICPrevScaledInput=0  ExternalReset=none  TrackingMode=off  Kt=1  LimitOutput=on  SatLimitsSource=internal  UpperSaturationLimit=S*C11*(2*(max_pot-u0))  LowerSaturationLimit=-S*C11*(2*(max_pot-u0))  LinearizeAsGain=on  AntiWindupMode=clamping  Kb=1  LimitIntegrator=off  UpperIntegratorSaturationLimit=inf  LowerIntegratorSaturationLimit=-inf  POutMin=[]  POutMax=[]  IOutMin=[]  IOutMax=[]  DOutMin=[]  DOutMax=[]  NOutMin=[]  NOutMax=[]  SumOutMin=[]  SumOutMax=[]  SaturationOutMin=[]  SaturationOutMax=[]  PParamMin=[]  PParamMax=[]  IParamMin=[]  IParamMax=[]  DParamMin=[]  DParamMax=[]  NParamMin=[]  NParamMax=[]  KbParamMin=[]  KbParamMax=[]  KtParamMin=[]  KtParamMax=[]  KbOutMin=[]  KbOutMax=[]  KtOutMin=[]  KtOutMax=[]  IntegratorOutMin=[]  IntegratorOutMax=[]  FilterOutMin=[]  FilterOutMax=[]  SumI1OutMin=[]  SumI1OutMax=[]  SumI2OutMin=[]  SumI2OutMax=[]  SumI3OutMin=[]  SumI3OutMax=[]  SumI4OutMin=[]  SumI4OutMax=[]  SumDOutMin=[]  SumDOutMax=[]  DifferentiatorOutMin=[]  DifferentiatorOutMax=[]  FilterDiffOutCoefMin=[]  FilterDiffOutCoefMax=[]  ReciprocalOutMin=[]  ReciprocalOutMax=[]  SumDenOutMin=[]  SumDenOutMax=[]  SumNumOutMin=[]  SumNumOutMax=[]  DivideOutMin=[]  DivideOutMax=[]  UdiffTsProdOutMin=[]  UdiffTsProdOutMax=[]  NTsProdOutMin=[]  NTsProdOutMax=[]  UintegralTsProdOutMin=[]  UintegralTsProdOutMax=[]  UngainTsProdOutMin=[]  UngainTsProdOutMax=[]  ClampingZeroOutDataTypeStr=Inherit: Inherit via back propagation  ClampingZeroOutMin=[]  ClampingZeroOutMax=[]  FilterDenConstantOutDataTypeStr=Inherit: Inherit via back propagation  FilterDenConstantOutMin=[]  FilterDenConstantOutMax=[]  PCopyOutDataTypeStr=Inherit: Inherit via back propagation  PCopyOutMin=[]  PCopyOutMax=[]  NCopyOutDataTypeStr=Inherit: Inherit via back propagation  NCopyOutMin=[]  NCopyOutMax=[]  IntegratorContinuousStateAttributes=''  IntegratorStateMustResolveToSignalObject=off  IntegratorRTWStateStorageClass=Auto  FilterContinuousStateAttributes=''  FilterStateMustResolveToSignalObject=off  FilterRTWStateStorageClass=Auto  ParallelPVariant=InternalParameters  IdealPVariant=Disabled  IVariant=InternalParameters  DVariant=InternalParameters  IntegratorVariant=Discrete  SatVariant=Enabled  AWVariant=DiscClampingParallel  PCopyVariant=Disabled  TRVariant=Disabled  FdbkBlocksVariant=Forward  IdealPFdbkVariant=Disabled  SatFdbkVariant=Disabled  DerivativeFilterVariant=ForwardEulerFilter  NVariant=InternalParameters  NCopyVariant=Disabled  FilterICVariant=InternalICsFilter  IntegratorICVariant=InternalICs  ExternalResetVariant=Disabled  TRSumVariant=Passthrough  SumFdbkVariant=Disabled  SumVariant=Sum_PID  TsampFilterVariant=InternalTs  TsampNgainVariant=Passthrough  TsampIntegralVariant=Disabled_SignalSpec  ExternalSaturationOutDataTypeStr=Inherit: Same as second input  DerivativeSourceVariant=ErrorSignal  PreIntVariant=InternalPreInt
  Pitch FF Gain : Gain  Gain=0
  Sum1 : Sum  Inputs=+-|
  Sum2 : Sum  Inputs=+|+
  Transfer Fcn : TransferFcn  Denominator=[0.05 1]
  Unit Delay : UnitDelay  InitialCondition=X0(8)  SampleTime=-1  HasFrameUpgradeWarning=on
  Pitch Axis Output : Outport
  wires:
  Pitch FF Gain/1 -> Sum2/1
  Pitch Rate Estimate/1 -> Sum1/2
  Transfer Fcn/1 -> Pitch FF Gain/1
  Sum2/1 -> Pitch Axis Output/1  "Pitch Axis Output"
  Pitch Rate SP/1 -> Unit Delay/1, Sum1/1
  Unit Delay/1 -> Transfer Fcn/1
  PID Controller1/1 -> Sum2/2  "Pitch PID Output"
  Sum1/1 -> PID Controller1/1  "Pitch Rate Error"

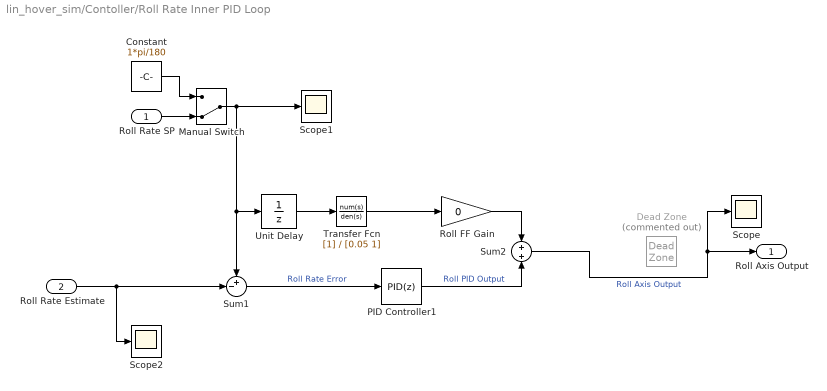
== system lin_hover_sim/Contoller/Roll Rate Inner PID Loop ==
  Roll Rate SP : Inport
  Roll Rate Estimate : Inport  Port=2
  Constant : Constant  Value=1*pi/180
  Dead Zone : DeadZone  Commented=on  LowerValue=-S*C11*(100)  UpperValue=S*C11*(100)
  Manual Switch : ManualSwitch  CurrentSetting=0
  PID Controller1 : slpidlib/PID Controller  Controller=PID  Form=Parallel  TimeDomain=Discrete-time  UseExternalTs=off  SampleTime=Ts  IntegratorMethod=Forward Euler  FilterMethod=Forward Euler  ControllerParametersSource=internal  P=roll_P  I=roll_I  UseKiTs=off  D=roll_D  UseExternalDerivativeSource=off  N=40  UseFilter=on  TunerSelectOption=Transfer Function Based (PID Tuner App)  InitialConditionSource=internal  InitialConditionForIntegrator=Xref(10) - X0(10)  InitialConditionForFilter=0  DifferentiatorICPrevScaledInput=0  ExternalReset=none  TrackingMode=off  Kt=1  LimitOutput=on  SatLimitsSource=internal  UpperSaturationLimit=S*C11*(2*(max_pot-u0))  LowerSaturationLimit=-S*C11*(2*(max_pot-u0))  LinearizeAsGain=on  AntiWindupMode=clamping  Kb=1  LimitIntegrator=off  UpperIntegratorSaturationLimit=inf  LowerIntegratorSaturationLimit=-inf  POutMin=[]  POutMax=[]  IOutMin=[]  IOutMax=[]  DOutMin=[]  DOutMax=[]  NOutMin=[]  NOutMax=[]  SumOutMin=[]  SumOutMax=[]  SaturationOutMin=[]  SaturationOutMax=[]  PParamMin=[]  PParamMax=[]  IParamMin=[]  IParamMax=[]  DParamMin=[]  DParamMax=[]  NParamMin=[]  NParamMax=[]  KbParamMin=[]  KbParamMax=[]  KtParamMin=[]  KtParamMax=[]  KbOutMin=[]  KbOutMax=[]  KtOutMin=[]  KtOutMax=[]  IntegratorOutMin=[]  IntegratorOutMax=[]  FilterOutMin=[]  FilterOutMax=[]  SumI1OutMin=[]  SumI1OutMax=[]  SumI2OutMin=[]  SumI2OutMax=[]  SumI3OutMin=[]  SumI3OutMax=[]  SumI4OutMin=[]  SumI4OutMax=[]  SumDOutMin=[]  SumDOutMax=[]  DifferentiatorOutMin=[]  DifferentiatorOutMax=[]  FilterDiffOutCoefMin=[]  FilterDiffOutCoefMax=[]  ReciprocalOutMin=[]  ReciprocalOutMax=[]  SumDenOutMin=[]  SumDenOutMax=[]  SumNumOutMin=[]  SumNumOutMax=[]  DivideOutMin=[]  DivideOutMax=[]  UdiffTsProdOutMin=[]  UdiffTsProdOutMax=[]  NTsProdOutMin=[]  NTsProdOutMax=[]  UintegralTsProdOutMin=[]  UintegralTsProdOutMax=[]  UngainTsProdOutMin=[]  UngainTsProdOutMax=[]  ClampingZeroOutDataTypeStr=Inherit: Inherit via back propagation  ClampingZeroOutMin=[]  ClampingZeroOutMax=[]  FilterDenConstantOutDataTypeStr=Inherit: Inherit via back propagation  FilterDenConstantOutMin=[]  FilterDenConstantOutMax=[]  PCopyOutDataTypeStr=Inherit: Inherit via back propagation  PCopyOutMin=[]  PCopyOutMax=[]  NCopyOutDataTypeStr=Inherit: Inherit via back propagation  NCopyOutMin=[]  NCopyOutMax=[]  IntegratorContinuousStateAttributes=''  IntegratorStateMustResolveToSignalObject=off  IntegratorRTWStateStorageClass=Auto  FilterContinuousStateAttributes=''  FilterStateMustResolveToSignalObject=off  FilterRTWStateStorageClass=Auto  ParallelPVariant=InternalParameters  IdealPVariant=Disabled  IVariant=InternalParameters  DVariant=InternalParameters  IntegratorVariant=Discrete  SatVariant=Enabled  AWVariant=DiscClampingParallel  PCopyVariant=Disabled  TRVariant=Disabled  FdbkBlocksVariant=Forward  IdealPFdbkVariant=Disabled  SatFdbkVariant=Disabled  DerivativeFilterVariant=ForwardEulerFilter  NVariant=InternalParameters  NCopyVariant=Disabled  FilterICVariant=InternalICsFilter  IntegratorICVariant=InternalICs  ExternalResetVariant=Disabled  TRSumVariant=Passthrough  SumFdbkVariant=Disabled  SumVariant=Sum_PID  TsampFilterVariant=InternalTs  TsampNgainVariant=Passthrough  TsampIntegralVariant=Disabled_SignalSpec  ExternalSaturationOutDataTypeStr=Inherit: Same as second input  DerivativeSourceVariant=ErrorSignal  PreIntVariant=InternalPreInt
  Roll FF Gain : Gain  Gain=0
  Scope : Scope
      settings: ActiveDisplayYMinimum=-1  ActiveDisplayYMaximum=1  DataLoggingVariableName=ScopeData5
  Scope1 : Scope
      settings: ActiveDisplayYMinimum=-3.8107976644369375  ActiveDisplayYMaximum=0.42890267258524473  DataLoggingVariableName=ScopeData7
  Scope2 : Scope
      settings: ActiveDisplayYMinimum=-0.22955859178227503  ActiveDisplayYMaximum=0.06191165222621095  DataLoggingVariableName=ScopeData8
  Sum1 : Sum  Inputs=+-|
  Sum2 : Sum  Inputs=+|+
  Transfer Fcn : TransferFcn  Denominator=[0.05 1]
  Unit Delay : UnitDelay  InitialCondition=X0(7)  SampleTime=-1  HasFrameUpgradeWarning=on
  Roll Axis Output : Outport
  wires:
  Roll FF Gain/1 -> Sum2/1
  Roll Rate Estimate/1 -> Scope2/1, Sum1/2
  Transfer Fcn/1 -> Roll FF Gain/1
  PID Controller1/1 -> Sum2/2  "Roll PID Output"
  Sum1/1 -> PID Controller1/1  "Roll Rate Error"
  Unit Delay/1 -> Transfer Fcn/1
  Constant/1 -> Manual Switch/1
  Manual Switch/1 -> Scope1/1, Unit Delay/1, Sum1/1
  Roll Rate SP/1 -> Manual Switch/2
  Sum2/1 -> Scope/1, Roll Axis Output/1  "Roll Axis Output"

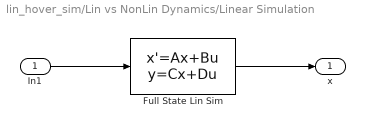
== system lin_hover_sim/Lin vs NonLin Dynamics/Linear Simulation ==
  In1 : Inport
  Full State Lin Sim : StateSpace  A=A  B=B  C=eye(12)  D=zeros(12,4)  InitialCondition=X0
  x : Outport
  wires:
  In1/1 -> Full State Lin Sim/1
  Full State Lin Sim/1 -> x/1

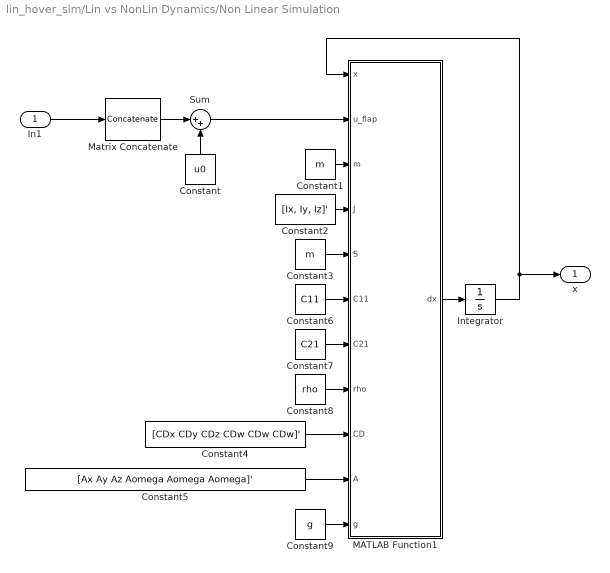
== system lin_hover_sim/Lin vs NonLin Dynamics/Non Linear Simulation ==
  In1 : Inport
  Constant : Constant  Value=u0
  Constant1 : Constant  Value=m
  Constant2 : Constant  Value=[Ix, Iy, Iz]'
  Constant3 : Constant  Value=m
  Constant4 : Constant  Value=[CDx CDy CDz CDw CDw CDw]'
  Constant5 : Constant  Value=[Ax Ay Az Aomega Aomega Aomega]'
  Constant6 : Constant  Value=C11
  Constant7 : Constant  Value=C21
  Constant8 : Constant  Value=rho
  Constant9 : Constant  Value=g
  Integrator : Integrator  InitialCondition=X0
  MATLAB Function1 : MATLAB Function  TreatAsAtomicUnit=on
  Matrix Concatenate : Concatenate  NumInputs=1
  Sum : Sum  Inputs=|++
  x : Outport
  wires:
  MATLAB Function1/1(dx) -> Integrator/1
  Integrator/1 -> MATLAB Function1/1(x), x/1
  In1/1 -> Matrix Concatenate/1
  Sum/1 -> MATLAB Function1/2(u_flap)
  Constant/1 -> Sum/2
  Constant1/1 -> MATLAB Function1/3(m)
  Constant2/1 -> MATLAB Function1/4(J)
  Constant3/1 -> MATLAB Function1/5(S)
  Constant5/1 -> MATLAB Function1/10(A)
  Constant7/1 -> MATLAB Function1/7(C21)
  Constant8/1 -> MATLAB Function1/8(rho)
  Constant6/1 -> MATLAB Function1/6(C11)
  Constant4/1 -> MATLAB Function1/9(CD)
  Constant9/1 -> MATLAB Function1/11(g)
  Matrix Concatenate/1 -> Sum/1

== matlab function lin_hover_sim/State Estimation/My Gyro LPF ==
  data: x input; xlpf output; gyro_alpha input
function xlpf = lpf(x,gyro_alpha)

persistent prevx_gyro firstrun_gyro

if isempty(firstrun_gyro)
    prevx_gyro = x;
    firstrun_gyro = 1;
end

xlpf = (1-gyro_alpha)*prevx_gyro + gyro_alpha*x;

prevx_gyro = xlpf;

end

== matlab function lin_hover_sim/Contoller/MATLAB Function ==
  data: u input; y output; C11 input; S input; k_tau input
function y = mix_quadflapper(u, C11, S, k_tau)
% u in this function is 
% [ Thrust command, 
%   roll moment command, 
%   pitch moment command, 
%   yaw moment command   ]

    if any(~isfinite(u))
    error('Mixer input contains NaN/Inf');
    end
    % Collective per-motor increment (note sign per your B row 6)
    uT = -u(1)/(4*(C11));

    % Roll and pitch differential components
    uR = u(2)/(2*S*C11);   % makes (du4 - du2) = taux/(S*C11)
    uP = u(3)/(2*S*C11);   % makes (du1 - du3) = tauy/(S*C11)

    % Yaw component (if available)
    if abs(k_tau) < 1e-12
        uY = 0;  % no yaw authority modeled
    else
        uY = u(4)/(4*k_tau); % makes (du1 - du2 + du3 - du4) = tauz/k_tau
    end
    
    
    du1 = uT + uP + uY;
    du2 = uT - uR - uY;
    du3 = uT - uP + uY;
    du4 = uT + uR - uY;

    y = [du1; du2; du3; du4]; % commanded change in pot value

    
end

== matlab function lin_hover_sim/State Estimation/My Accel LPF ==
  data: x input; xlpf output; accel_alpha input
function xlpf = lpf(x, accel_alpha)

persistent prevx_accel firstrun_accel

if isempty(firstrun_accel)
    prevx_accel = x;
    firstrun_accel = 1;
end

xlpf = (1-accel_alpha)*prevx_accel + accel_alpha*x;

prevx_accel = xlpf;

end

== matlab function lin_hover_sim/State Estimation/MATLAB Function ==
  data: gyro input; eul output; omega_out output; accel input; Ts input; Kp input; Ki input; eul0 input; b_hat_out output; q_out output
function [eul, omega_out, b_hat_out, q_out] = mahony_explicit_accel_only_simulink(gyro, accel, Ts, Kp, Ki, eul0)
%#codegen
% mahony_explicit_accel_only_simulink
%
% Simulink MATLAB Function block version of Mahony explicit complementary
% filter using gyro + accelerometer only.
%
% Inputs:
%   gyro  = [p; q; r] body rates in rad/s
%   accel = [ax; ay; az] accelerometer measurement
%   Ts    = sample time [s]
%   Kp    = proportional correction gain
%   Ki    = integral/bias correction gain
%   eul0  = [roll0; pitch0; yaw0] initial attitude in radians
%   reset = reset/reinitialize flag, boolean or 0/1
%
% Outputs:
%   eul       = [roll; pitch; yaw] in radians
%   b_hat_out = estimated gyro bias [rad/s]
%   q_out     = current quaternion [qw; qx; qy; qz]
%
% Notes:
%   - Roll and pitch are corrected using accelerometer.
%   - Yaw is only gyro-integrated and will drift with accel-only correction.
%   - This assumes level stationary accel is approximately [0; 0; +g].
%   - Quaternion convention is [qw; qx; qy; qz].

persistent q b_hat initialized

if isempty(initialized)
    q = eul321_to_quat(eul0(1), eul0(2), eul0(3));
    b_hat = zeros(3,1);
    initialized = true;
end

% if reset ~= 0
%     q = eul321_to_quat(eul0(1), eul0(2), eul0(3));
%     b_hat = zeros(3,1);
%     reset = 0;          % make reset false after initialization
% end

% -----------------------------
% Measurement correction
% -----------------------------
omega_mes = zeros(3,1);

accNorm = sqrt(accel(1)^2 + accel(2)^2 + accel(3)^2);

if accNorm > 1e-9

    % Measured gravity direction in body frame
    v = accel / accNorm;

    qw = q(1);
    qx = q(2);
    qy = q(3);
    qz = q(4);

    % Estimated gravity direction in body frame from current attitude
    %
    % This assumes level stationary accel is approximately [0; 0; +g].
    v_hat = [ ...
        2.0*(qx*qz - qw*qy);
        2.0*(qw*qx + qy*qz);
        qw*qw - qx*qx - qy*qy + qz*qz ];

    % Mahony explicit complementary filter innovation
    omega_mes = cross3(v, v_hat);

    % If your attitude correction diverges instead of converging,
    % flip the sign by using this instead:
    % omega_mes = cross3(v_hat, v);

end

% -----------------------------
% Bias estimate update
% -----------------------------
% This estimates gyro bias in observable directions.
% With accel-only correction, yaw bias is not observable.
b_hat = b_hat - Ki * omega_mes * Ts;

% Corrected gyro
omega = gyro - b_hat + Kp * omega_mes;

%Output Corrected rates !!!!!!!!!!!!!!!!!!!!!!!!!!!!!!!!!!!!!!!!!!!!!!!!
omega_out = gyro - b_hat; % These are the corrected body angular rates that can be used for rate control outside of this estimator

% -----------------------------
% Quaternion propagation using corrected omega
% -----------------------------
qw = q(1);
qx = q(2);
qy = q(3);
qz = q(4);

p = omega(1);
qrate = omega(2);
r = omega(3);

qdot = 0.5 * [ ...
    -qx*p - qy*qrate - qz*r;
     qw*p + qy*r     - qz*qrate;
     qw*qrate - qx*r + qz*p;
     qw*r + qx*qrate - qy*p ];

q = q + qdot * Ts;

% Normalize quaternion
qnorm = sqrt(q(1)^2 + q(2)^2 + q(3)^2 + q(4)^2);

if qnorm > 1e-12
    q = q / qnorm;
else
    q = eul321_to_quat(eul0(1), eul0(2), eul0(3));
    b_hat = zeros(3,1);
end

% -----------------------------
% Quaternion to Euler angles
% -----------------------------
qw = q(1);
qx = q(2);
qy = q(3);
qz = q(4);

roll = atan2( ...
    2.0*(qw*qx + qy*qz), ...
    1.0 - 2.0*(qx*qx + qy*qy) );

sinPitch = 2.0*(qw*qy - qz*qx);

if sinPitch > 1.0
    sinPitch = 1.0;
elseif sinPitch < -1.0
    sinPitch = -1.0;
end

pitch = asin(sinPitch);

yaw = atan2( ...
    2.0*(qw*qz + qx*qy), ...
    1.0 - 2.0*(qy*qy + qz*qz) );

% Output Euler Angles !!!!!!!!!!!!!!!!!!!!!!!!!!!!!!!!!!!!!!!!!!!!!!!!
eul = [roll; pitch; yaw];

% Output Bias Estimate and Quaternion Estimate !!!!!!!!!!!!!!!!!!!!!!!!!!!!!!!!!!!!!!!!!!!!!!!!
b_hat_out = b_hat;
q_out = q;

end


function q = eul321_to_quat(roll, pitch, yaw)
% eul321_to_quat
%
% Converts 3-2-1 yaw-pitch-roll Euler angles to quaternion [qw; qx; qy; qz].
%
% roll  = phi
% pitch = theta
% yaw   = psi

cr = cos(0.5*roll);
sr = sin(0.5*roll);

cp = cos(0.5*pitch);
sp = sin(0.5*pitch);

cy = cos(0.5*yaw);
sy = sin(0.5*yaw);

qw = cy*cp*cr + sy*sp*sr;
qx = cy*cp*sr - sy*sp*cr;
qy = cy*sp*cr + sy*cp*sr;
qz = sy*cp*cr - cy*sp*sr;

q = [qw; qx; qy; qz];

% Normalize for safety
qnorm = sqrt(qw*qw + qx*qx + qy*qy + qz*qz);
if qnorm > 1e-12
    q = q / qnorm;
else
    q = [1; 0; 0; 0];
end

end


function c = cross3(a, b)
% cross3
%
% Manual 3D cross product for code generation clarity.

c = [ ...
    a(2)*b(3) - a(3)*b(2);
    a(3)*b(1) - a(1)*b(3);
    a(1)*b(2) - a(2)*b(1) ];

end

== matlab function lin_hover_sim/MATLAB Function ==
  data: x input; accel_ideal output; du input; gyro_ideal output; m parameter; g parameter; C11 parameter; Xu parameter; Yv parameter; Zw parameter; noise_true parameter
function [accel_ideal, gyro_ideal] = ideal_imu_measurements( ...
    x, du, m, g, C11, Xu, Yv, Zw, noise_true)
%#codegen
%
% x  = [x y z u v w phi theta psi p q r]'
% du = [du1 du2 du3 du4]' motor/flapper increments from hover trim
%
% Body/NED convention:
%   body x forward
%   body y right
%   body z down
%   thrust acts in negative body-z
%
% Output:
%   accel_ideal = ideal accelerometer specific force [m/s^2]
%                 level stationary hover -> [0; 0; -g]
%   gyro_ideal  = ideal gyro measurement [rad/s]

% -----------------------------
% Extract states
% -----------------------------
u_b = x(4);
v_b = x(5);
w_b = x(6);

phi   = x(7);   % roll
theta = x(8);   % pitch
% psi not needed for gravity projection into body z-down accel convention

p = x(10);
q = x(11);
r = x(12);

% -----------------------------
% Nonlinear gravity / specific-force direction
% -----------------------------
% Ideal accelerometer at rest measures specific force opposite gravity.
%
% For body z down:
%   level stationary hover -> [0; 0; -g]
%
% Nonlinear version:
accel_gravity = [ g*sin(theta);
                 -g*sin(phi)*cos(theta);
                 -g*cos(phi)*cos(theta)];

% -----------------------------
% Simple external acceleration terms
% -----------------------------

% Linear drag/damping accelerations from your plant model
a_drag = [-(Xu/m)*u_b;
          -(Yv/m)*v_b;
          -(Zw/m)*w_b];

% Incremental thrust acceleration from your B matrix
% Since hover thrust is already represented by accel_gravity = [0;0;-g]
% only add incremental thrust from du here.
a_thrust = [0;
            0;
           -(C11/m)*sum(du)];

% -----------------------------
% Ideal accel and gyro outputs
% -----------------------------
accel_ideal = accel_gravity + noise_true*a_drag + noise_true*a_thrust;

gyro_ideal = [p;
              q;
              r];

end

== matlab function lin_hover_sim/Lin vs NonLin Dynamics/Non Linear Simulation/MATLAB Function1 ==
  data: x input; dx output size=12; u_flap input; m input; J input; S input; C11 input; C21 input; rho input; CD input; A input; g input
function dx = nonlinearEOM(x,u_flap,m,J,S,C11,C21,rho,CD,A,g)
%#codegen
% x      = [x y z u v w phi theta psi p q r]'
% u_flap = absolute flapper commands [u1 u2 u3 u4]' [pot]
% J      = [Ix Iy Iz]'
% CD     = [CDx CDy CDz CDp CDq CDr]'
% A      = [Ax Ay Az Ap Aq Ar]'
% Body/inertial z positive down; 3-2-1 Euler angles

u=x(4); v=x(5); w=x(6); ph=x(7); th=x(8); ps=x(9);
p=x(10); q=x(11); r=x(12); Ix=J(1); Iy=J(2); Iz=J(3);

% Actual flapper thrusts, positive upward (-z body)
T = C11*u_flap + C21;

% Quadratic translational drag + total flapper thrust
F = -.5*rho*CD(1:3).*A(1:3).*abs([u;v;w]).*[u;v;w];
F(3) = F(3) - sum(T);

% Flapper moments + quadratic rotational drag
M = [S*(T(4)-T(2)); S*(T(1)-T(3)); 0] ...
    - .5*rho*CD(4:6).*A(4:6)*S^3.*abs([p;q;r]).*[p;q;r];

% Nonlinear translational dynamics
vd = F/m + [-g*sin(th); g*sin(ph)*cos(th); g*cos(ph)*cos(th)] ...
     - cross([p;q;r],[u;v;w]);

% Nonlinear rotational dynamics
wd = [(M(1)-(Iz-Iy)*q*r)/Ix;
      (M(2)-(Ix-Iz)*p*r)/Iy;
      (M(3)-(Iy-Ix)*p*q)/Iz];

% Exact 3-2-1 Euler-angle kinematics
E = [1 sin(ph)*tan(th) cos(ph)*tan(th);
     0 cos(ph)        -sin(ph);
     0 sin(ph)/cos(th) cos(ph)/cos(th)];

% Inertial-to-body DCM
C_bI = [cos(th)*cos(ps), cos(th)*sin(ps), -sin(th);
        sin(ph)*sin(th)*cos(ps)-cos(ph)*sin(ps), ...
        sin(ph)*sin(th)*sin(ps)+cos(ph)*cos(ps), sin(ph)*cos(th);
        cos(ph)*sin(th)*cos(ps)+sin(ph)*sin(ps), ...
        cos(ph)*sin(th)*sin(ps)-sin(ph)*cos(ps), cos(ph)*cos(th)];

% Full state derivative
dx = [C_bI'*[u;v;w]; vd; E*[p;q;r]; wd];
end
